simulink model "chap5_8sim"  (Simulink 8.1)
settings: Solver=ode3  StartTime=0  StopTime=20  FixedStep=0.01  RelTol=1e-3  AbsTol=1e-3
settings Model: Creator=liujk  LastModifiedBy=liujk  ExtModeTrigMode=oneshot  ExtModeArmWhenConnect=off
settings DataIOCC: LimitDataPoints=off  SignalLoggingName=sigsOut
settings OptimizationCC: BooleanDataType=off  ExpressionDepthLimit=128  InitFltsAndDblsToZero=on
settings DebuggingCC: SaveWithParameterizedLinksMsg=none  SignalResolutionControl=TryResolveAllWithWarning  SolverPrmCheckMsg=none  MultiTaskDSMMsg=warning  MultiTaskCondExecSysMsg=none  StrictBusMsg=None
settings HardwareCC: TargetIntDivRoundTo=Zero  TargetEndianess=LittleEndian  TargetHWDeviceType=MATLAB Host  ProdEqTarget=off
settings RTWCC: IncludeERTFirstTime=on
settings GRTTargetCC: TargetFcnLib=ansi_tfl_tmw.mat

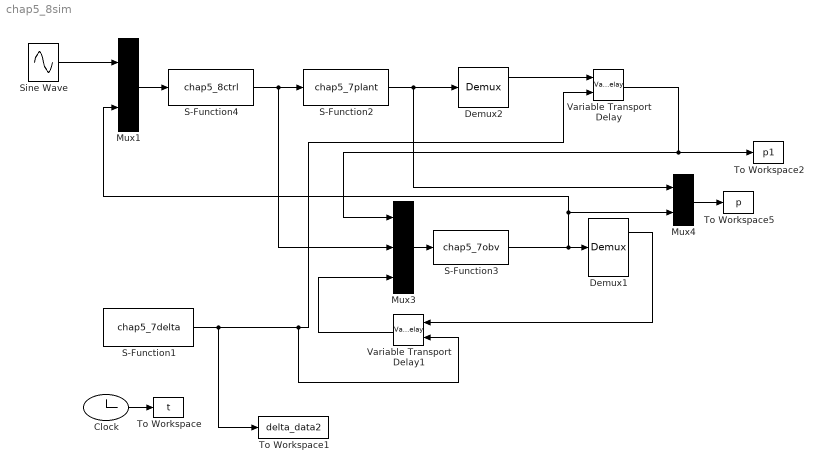
== system chap5_8sim ==
  Clock : Clock
  Demux1 : Demux  Outputs=2
  Demux2 : Demux  Outputs=2
  Mux1 : Mux  Inputs=2
  Mux3 : Mux  Inputs=3
  Mux4 : Mux  Inputs=2
  S-Function1 : S-Function  FunctionName=chap5_7delta  EnableBusSupport=off
  S-Function2 : S-Function  FunctionName=chap5_7plant  EnableBusSupport=off
  S-Function3 : S-Function  FunctionName=chap5_7obv  EnableBusSupport=off
  S-Function4 : S-Function  FunctionName=chap5_8ctrl  EnableBusSupport=off
  Sine Wave : Sin  SampleTime=0
  To Workspace : ToWorkspace  VariableName=t  SampleTime=-1
  To Workspace1 : ToWorkspace  VariableName=delta_data2  SampleTime=-1
  To Workspace2 : ToWorkspace  VariableName=p1  SampleTime=-1
  To Workspace5 : ToWorkspace  VariableName=p  SampleTime=-1
  Variable Transport Delay : VariableTransportDelay  MaximumDelay=10
  Variable Transport Delay1 : VariableTransportDelay  MaximumDelay=10
  wires:
  Clock/1 -> To Workspace/1
  Mux3/1 -> S-Function3/1
  Variable Transport Delay1/1 -> Mux3/3
  S-Function2/1 -> Mux4/1, Demux2/1
  Variable Transport Delay/1 -> Mux3/1, To Workspace2/1
  Mux4/1 -> To Workspace5/1
  S-Function3/1 -> Mux4/2, Mux1/2, Demux1/1
  Demux1/1 -> Variable Transport Delay1/1
  S-Function1/1 -> Variable Transport Delay/2, Variable Transport Delay1/2, To Workspace1/1
  Demux2/1 -> Variable Transport Delay/1
  S-Function4/1 -> S-Function2/1, Mux3/2
  Mux1/1 -> S-Function4/1
  Sine Wave/1 -> Mux1/1
